simulink model "Assignment_2_model"  (R2022a)
settings: Solver=FixedStepDiscrete  StartTime=0.0  StopTime=360  FixedStep=1  RelTol=1e-3
values from neighbouring files (symbols this model uses):
  salary_increase_rate = combinations(2,i)    [Assignment_2_tests.m]
undefined symbols (not defined in the file or in its folder): DiscIntNeverNeededParam, interest
settings Model: Creator=h17163  LastModifiedBy=anton
settings SolverCC: AlgebraicLoopSolver=TrustRegion
settings DataIOCC: ReturnWorkspaceOutputs=off
settings DebuggingCC: UnconnectedInputMsg=warning  UnconnectedOutputMsg=warning  UnconnectedLineMsg=warning  SFMachineParentedDataDiag=warning  ArithmeticOperatorsInVariantConditions=warning
settings SFSimCC: SimUseLocalCustomCode=off  CustomCodeUndefinedFunction=UseInterfaceOnly
settings RTWCC: RTWUseLocalCustomCode=off

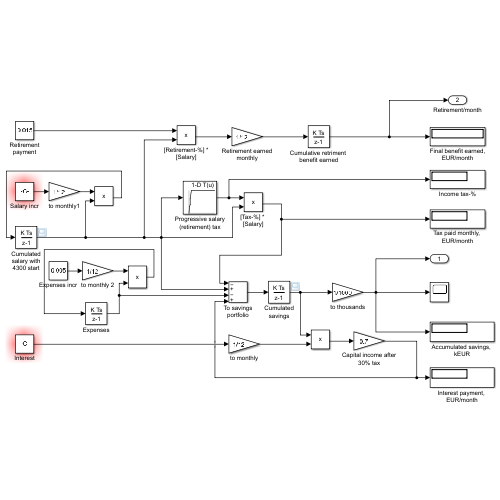
[thumbnail: Simulink's stored preview of the top-level diagram]
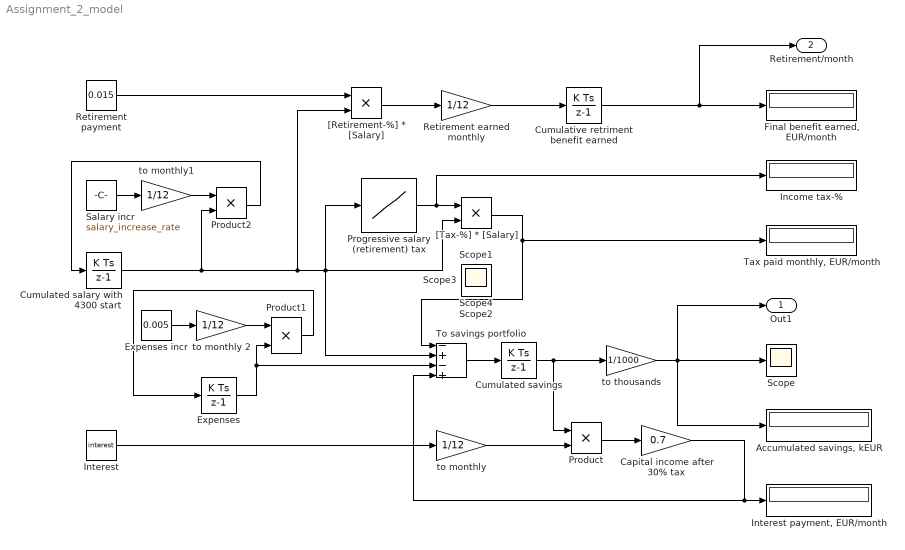
== system Assignment_2_model ==
  "Accumulated savings, kEUR" : Display
  Capital income after 30% tax : Gain  Gain=0.7
  Cumulated salary with 4300 start : DiscreteIntegrator  InitialCondition=4300  SampleTime=-1  ICPrevOutput=DiscIntNeverNeededParam  ICPrevScaledInput=DiscIntNeverNeededParam
  Cumulated savings : DiscreteIntegrator  SampleTime=-1  ICPrevOutput=DiscIntNeverNeededParam  ICPrevScaledInput=DiscIntNeverNeededParam
  Cumulative retriment benefit earned : DiscreteIntegrator  SampleTime=-1  ICPrevOutput=DiscIntNeverNeededParam  ICPrevScaledInput=DiscIntNeverNeededParam
  Expenses : DiscreteIntegrator  InitialCondition=3200  SampleTime=-1  ICPrevOutput=DiscIntNeverNeededParam  ICPrevScaledInput=DiscIntNeverNeededParam
  Expenses incr : Constant  Value=0.005
  "Final benefit earned, EUR/month" : Display
  Income tax-% : Display
  Interest : Constant  Value=interest
  "Interest payment, EUR/month" : Display
  Product : Product
  Product1 : Product
  Product2 : Product
  Progressive salary (retirement) tax : Lookup_n-D  NumberOfTableDimensions=1  BreakpointsForDimension1=[1000, 3000, 5000, 7000, 10000, 100000]  Table=[0, .17, .22, .37, .58, .58]  InternalRulePriority=Speed  RndMeth=Simplest
  Retirement payment : Constant  Value=0.015
  Retirement earned monthly : Gain  Gain=1/12
  Salary incr : Constant  Value=salary_increase_rate
  Scope{,1..4} (5 alike) : Scope
  "Tax paid monthly, EUR/month" : Display
  To savings portfolio : Sum  Inputs=-+-+
  "[Retirement-%] * [Salary]" : Product
  "[Tax-%] * [Salary]" : Product
  to monthly : Gain  Gain=1/12
  to monthly 2 : Gain  Gain=1/12
  to monthly1 : Gain  Gain=1/12
  to thousands : Gain  Gain=1/1000
  Out1 : Outport
  Retirement/month : Outport  Port=2
  wires:
  Expenses/1 -> To savings portfolio/3, Product1/2
  To savings portfolio/1 -> Cumulated savings/1
  to thousands/1 -> Out1/1, Scope/1, "Accumulated savings, kEUR"/1
  Interest/1 -> to monthly/1
  Cumulated savings/1 -> to thousands/1, Product/1
  to monthly/1 -> Product/2
  Progressive salary (retirement) tax/1 -> "[Tax-%] * [Salary]"/1, Income tax-%/1
  "[Tax-%] * [Salary]"/1 -> To savings portfolio/1, "Tax paid monthly, EUR/month"/1
  Retirement payment/1 -> "[Retirement-%] * [Salary]"/1
  "[Retirement-%] * [Salary]"/1 -> Retirement earned monthly/1
  Cumulative retriment benefit earned/1 -> Retirement/month/1, "Final benefit earned, EUR/month"/1
  Retirement earned monthly/1 -> Cumulative retriment benefit earned/1
  Product/1 -> Capital income after 30% tax/1
  Capital income after 30% tax/1 -> To savings portfolio/4, "Interest payment, EUR/month"/1
  Cumulated salary with 4300 start/1 -> Product2/2, To savings portfolio/2, "[Tax-%] * [Salary]"/2, Progressive salary (retirement) tax/1, "[Retirement-%] * [Salary]"/2
  Salary incr/1 -> to monthly1/1
  to monthly1/1 -> Product2/1
  Product2/1 -> Cumulated salary with 4300 start/1
  Expenses incr/1 -> to monthly 2/1
  to monthly 2/1 -> Product1/1
  Product1/1 -> Expenses/1
